simulink model "dubins_car"  (R2020b)
settings: Solver=VariableStepAuto  StartTime=0.0  StopTime=20  FixedStep=0.02  RelTol=1e-3
values from neighbouring files (symbols this model uses):
  err = phi * (x - pi_val)    [compute_error.m]    (also in concrete_controller.m = x - (P_1*xhat + P_2*uhat))
libraries: polylib x1
settings Model: Creator=swsmth  LastModifiedBy=swsmth
settings DataIOCC: ReturnWorkspaceOutputs=off
settings DebuggingCC: ArithmeticOperatorsInVariantConditions=warning
settings SFSimCC: SimUseLocalCustomCode=off  CustomCodeUndefinedFunction=UseInterfaceOnly
settings RTWCC: RTWUseLocalCustomCode=off

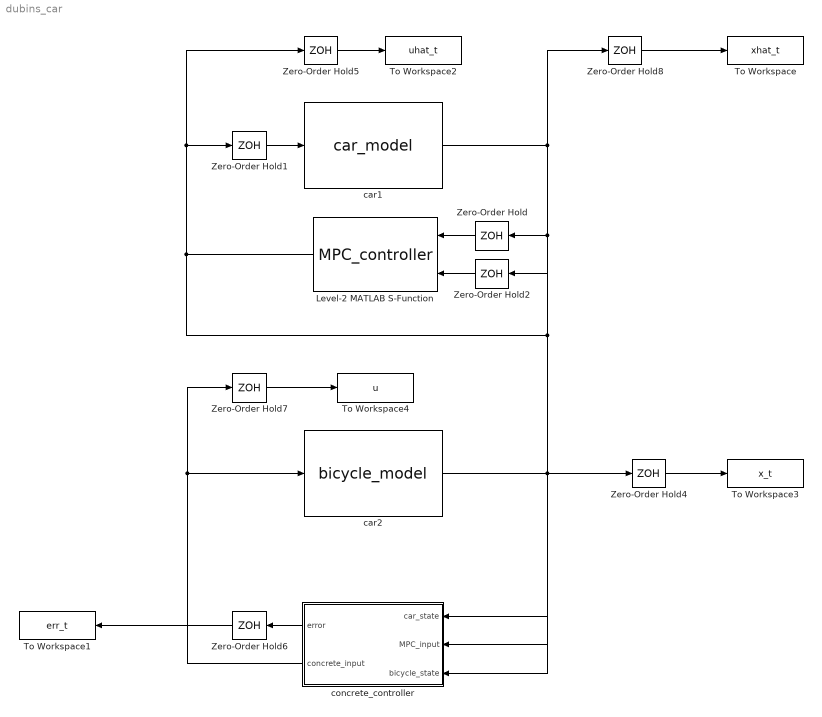
== system dubins_car ==
  Level-2 MATLAB S-Function : M-S-Function  FunctionName=MPC_controller
  To Workspace : ToWorkspace  VariableName=xhat_t  SampleTime=-1
  To Workspace1 : ToWorkspace  VariableName=err_t  SampleTime=-1
  To Workspace2 : ToWorkspace  VariableName=uhat_t  SampleTime=-1
  To Workspace3 : ToWorkspace  VariableName=x_t  SampleTime=-1
  To Workspace4 : ToWorkspace  VariableName=u  SampleTime=-1
  Zero-Order Hold{,1..2,4..8} (8 alike) : ZeroOrderHold  SampleTime=0.1
  car1 : M-S-Function  FunctionName=car_model
  car2 : M-S-Function  FunctionName=bicycle_model
  concrete_controller : Subsystem
  wires:
  Zero-Order Hold1/1 -> car1/1
  Level-2 MATLAB S-Function/1 -> concrete_controller/2(MPC_input), Zero-Order Hold2/1, Zero-Order Hold1/1, Zero-Order Hold5/1
  Zero-Order Hold5/1 -> To Workspace2/1
  car1/1 -> Zero-Order Hold8/1, Zero-Order Hold/1, concrete_controller/1(car_state)
  car2/1 -> Zero-Order Hold4/1, concrete_controller/3(bicycle_state)
  Zero-Order Hold7/1 -> To Workspace4/1
  Zero-Order Hold4/1 -> To Workspace3/1
  Zero-Order Hold2/1 -> Level-2 MATLAB S-Function/2
  Zero-Order Hold/1 -> Level-2 MATLAB S-Function/1
  Zero-Order Hold8/1 -> To Workspace/1
  concrete_controller/1(error) -> Zero-Order Hold6/1
  concrete_controller/2(concrete_input) -> car2/1, Zero-Order Hold7/1
  Zero-Order Hold6/1 -> To Workspace1/1

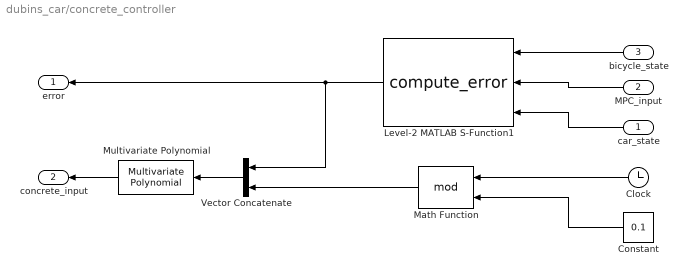
== system dubins_car/concrete_controller ==
  car_state : Inport
  MPC_input : Inport  Port=2
  bicycle_state : Inport  Port=3
  Clock : Clock
  Constant : Constant  Value=0.1
  Level-2 MATLAB S-Function1 : M-S-Function  FunctionName=compute_error
  Math Function : Math  Operator=mod  SaturateOnIntegerOverflow=on
  Multivariate Polynomial : polylib/Multivariate  Polynomial  p=p  x=[err; t]
  Vector Concatenate : Concatenate
  error : Outport
  concrete_input : Outport  Port=2
  wires:
  car_state/1 -> Level-2 MATLAB S-Function1/3
  MPC_input/1 -> Level-2 MATLAB S-Function1/2
  Level-2 MATLAB S-Function1/1 -> error/1, Vector Concatenate/1
  bicycle_state/1 -> Level-2 MATLAB S-Function1/1
  Vector Concatenate/1 -> Multivariate Polynomial/1
  Math Function/1 -> Vector Concatenate/2
  Clock/1 -> Math Function/1
  Constant/1 -> Math Function/2
  Multivariate Polynomial/1 -> concrete_input/1
